simulink model "rtwdemo_merge"  (Simulink 7.6)
settings: Solver=FixedStepDiscrete  StartTime=0.0  StopTime=10.0  RelTol=1e-3  SampleTimeConstraint=STIndependent
libraries: rtwdemowidgets x2
Description:
  | Temporary Variables for Merged Signals
settings Model: Creator=The MathWorks Inc.  CovMetricSettings=d  ExtModeAutoUpdateStatusClock=off
settings DataIOCC: SaveOutput=off  SaveTime=off  SignalLoggingName=sigsOut
settings OptimizationCC: InlineParams=on  InlineInvariantSignals=on  StateBitsets=on  DataBitsets=on  UseTempVars=on  EfficientFloat2IntCast=on  EfficientMapNaN2IntZero=off
settings DebuggingCC: CheckExecutionContextPreStartOutputMsg=on  CheckExecutionContextRuntimeOutputMsg=on  SolverPrmCheckMsg=none  StrictBusMsg=ErrorOnBusTreatedAsVector
settings HardwareCC: ProdIntDivRoundTo=Zero  ProdEndianess=LittleEndian  ProdHWDeviceType=Generic->32-bit Embedded Processor  TargetHWDeviceType=Generic->32-bit Embedded Processor
settings RTWCC: TLCOptions=-p0 -aWarnNonSaturatedBlocks=0  GenerateReport=on  RTWVerbose=off  ProcessScript=grt_make_rtw_hook  LaunchReport=on
settings CodeAppCC: ForceParamTrailComments=on
settings GRTTargetCC: TargetFcnLib=ansi_tfl_tmw.mat

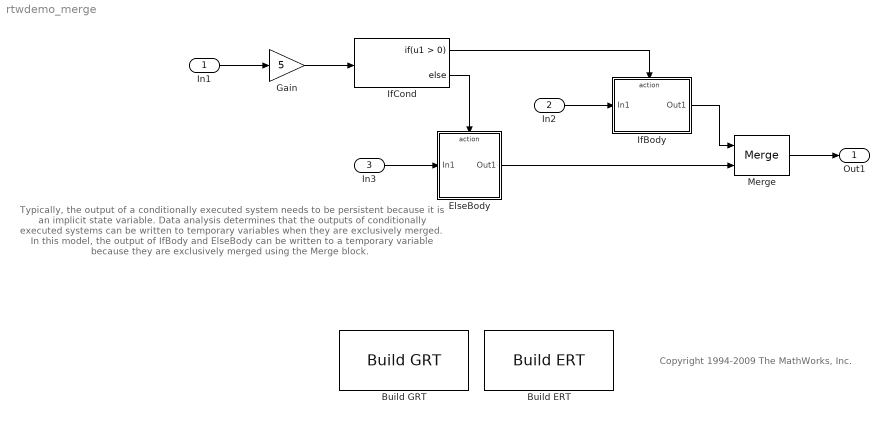
== system rtwdemo_merge ==
  note: Typically, the output of a conditionally executed system needs to be persistent because it is
      | an implicit state variable.  Data analysis determines that the outputs of conditionally executed
      | systems can be written to temporary variables when they are exclusively merged. In this model,
      | the output of IfBody and ElseBody can be written to a temporary variable because they are
      | exclusively merged using the Merge block.
  note: Copyright 1994-2009 The MathWorks, Inc.
  In1 : Inport  OutDataTypeStr=single  PortDimensions=1
  In2 : Inport  Port=2  OutDataTypeStr=single  PortDimensions=1
  In3 : Inport  Port=3  OutDataTypeStr=single  PortDimensions=1
  Build ERT : rtwdemowidgets/Build ERT  SystemSampleTime=-1  attrib_overrides={}
  Build GRT : rtwdemowidgets/Build GRT  SystemSampleTime=-1  attrib_overrides={}
  ElseBody : Subsystem  TreatAsAtomicUnit=on
  Gain : Gain  Gain=5  SaturateOnIntegerOverflow=on  OutDataTypeStr=Inherit: Same as input  ParamDataTypeStr=Inherit: Same as input
  IfBody : Subsystem  TreatAsAtomicUnit=on
  IfCond : If
  Merge : Merge
  Out1 : Outport
  wires:
  IfCond/1 -> IfBody/Action
  IfCond/2 -> ElseBody/Action
  In1/1 -> Gain/1
  In2/1 -> IfBody/1(In1)
  In3/1 -> ElseBody/1(In1)
  IfBody/1(Out1) -> Merge/1
  ElseBody/1(Out1) -> Merge/2
  Merge/1 -> Out1/1
  Gain/1 -> IfCond/1

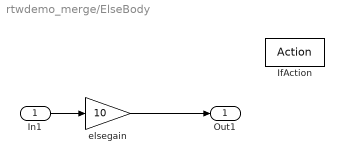
== system rtwdemo_merge/ElseBody ==
  In1 : Inport
  IfAction : ActionPort  ActionType=else
  elsegain : Gain  Gain=10  SaturateOnIntegerOverflow=on  OutDataTypeStr=Inherit: Same as input  ParamDataTypeStr=Inherit: Same as input
  Out1 : Outport
  wires:
  In1/1 -> elsegain/1
  elsegain/1 -> Out1/1

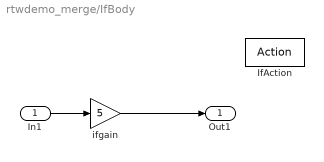
== system rtwdemo_merge/IfBody ==
  In1 : Inport
  IfAction : ActionPort  ActionType=then
  ifgain : Gain  Gain=5  SaturateOnIntegerOverflow=on  OutDataTypeStr=Inherit: Same as input  ParamDataTypeStr=Inherit: Same as input
  Out1 : Outport
  wires:
  In1/1 -> ifgain/1
  ifgain/1 -> Out1/1
